simulink model "model"  (R2020b)
settings: Solver=VariableStepAuto  StartTime=0.0  StopTime=10.0  RelTol=1e-3
undefined symbols (not defined in the file or in its folder): fmotors, frpy, fxyz
settings Model: Creator=Guillermo  LastModifiedBy=Guillermo

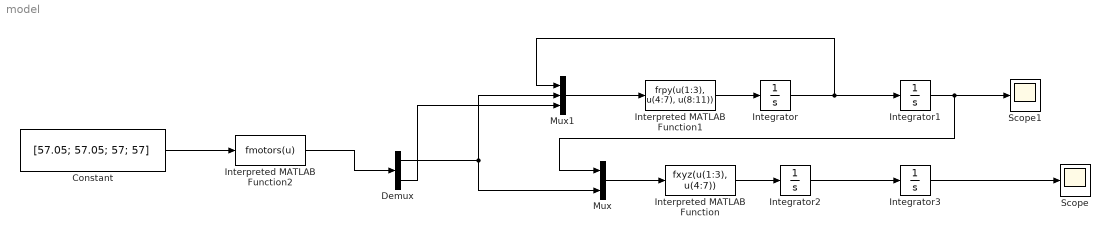
== system model ==
  Constant : Constant  Value=[57.05; 57.05; 57; 57]
  Demux : Demux  Outputs=2
  Integrator{,1..3} (4 alike) : Integrator
  Interpreted MATLAB Function : MATLABFcn  MATLABFcn=fxyz(u(1:3), u(4:7))
  Interpreted MATLAB Function1 : MATLABFcn  MATLABFcn=frpy(u(1:3), u(4:7), u(8:11))  OutputDimensions=3
  Interpreted MATLAB Function2 : MATLABFcn  MATLABFcn=fmotors(u)
  Mux : Mux  Inputs=2
  Mux1 : Mux  Inputs=3
  Scope : Scope
  Scope1 : Scope
  wires:
  Mux/1 -> Interpreted MATLAB Function/1
  Constant/1 -> Interpreted MATLAB Function2/1
  Interpreted MATLAB Function2/1 -> Demux/1
  Demux/1 -> Mux1/2, Mux/2
  Demux/2 -> Mux1/3
  Interpreted MATLAB Function1/1 -> Integrator/1
  Integrator/1 -> Mux1/1, Integrator1/1
  Integrator1/1 -> Scope1/1, Mux/1
  Interpreted MATLAB Function/1 -> Integrator2/1
  Integrator2/1 -> Integrator3/1
  Integrator3/1 -> Scope/1
  Mux1/1 -> Interpreted MATLAB Function1/1
